simulink model "Problem1_model"  (R2016a)
settings: Solver=VariableStepAuto  StartTime=0.0  StopTime=10.0  RelTol=1e-3
values from neighbouring files (symbols this model uses):
  theta1_path = planTraj(x2_i(1),x2_f(1),time)    [Problem1.m]    (also in Problem2.m)
  theta2_path = planTraj(x2_i(2),x2_f(2),time)    [Problem1.m]    (also in Problem2.m)
undefined symbols (not defined in the file or in its folder): x2_i
settings Model: Creator=nathaniel  LastModifiedBy=nathaniel
settings GRTTargetCC: GeneratePreprocessorConditionals=Use local settings

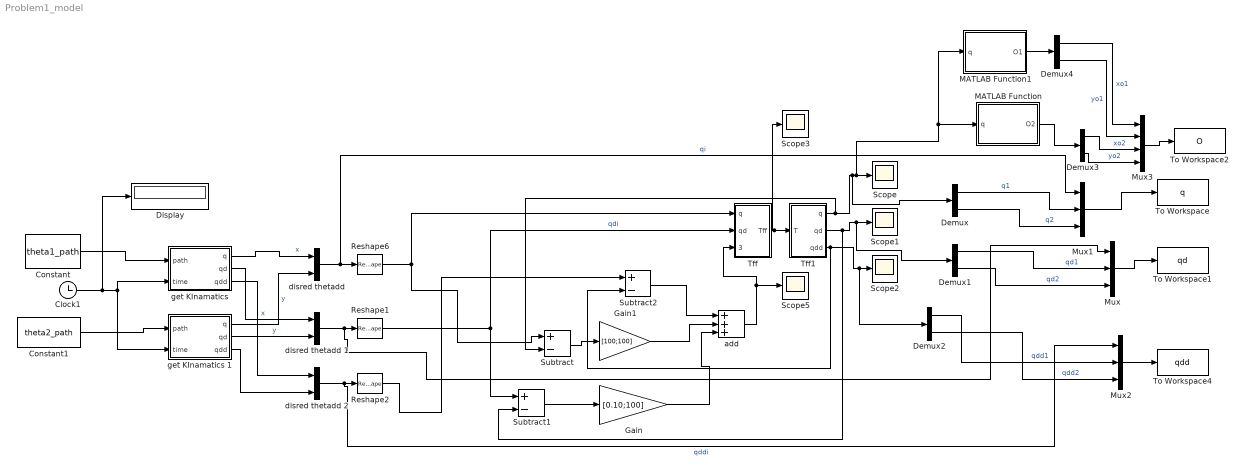
== system Problem1_model ==
  Clock1 : Clock
  Constant : Constant  Value=theta1_path
  Constant1 : Constant  Value=theta2_path
  Demux{,1..4} (5 alike) : Demux  Outputs=2
  Display : Display
  Gain : Gain  Gain=[0.10;100]
  Gain1 : Gain  Gain=[100;100]
  MATLAB Function : MATLAB Function  TreatAsAtomicUnit=on
  MATLAB Function1 : MATLAB Function  TreatAsAtomicUnit=on
  Mux : Mux  Inputs=3
  Mux1 : Mux  Inputs=3
  Mux2 : Mux  Inputs=3
  Mux3 : Mux
  Reshape1 : Reshape  OutputDimensionality=Column vector (2-D)
  Reshape2 : Reshape  OutputDimensionality=Column vector (2-D)
  Reshape6 : Reshape  OutputDimensionality=Column vector (2-D)
  Scope{,1..3,5} (5 alike) : Scope
  Subtract : Sum  Inputs=+-
  Subtract1 : Sum  Inputs=+-
  Subtract2 : Sum  Inputs=+-
  Tff : Subsystem
  Tff1 : Subsystem
  To Workspace : ToWorkspace  VariableName=q  SampleTime=-1
  To Workspace1 : ToWorkspace  VariableName=qd  SampleTime=-1
  To Workspace2 : ToWorkspace  VariableName=O  SampleTime=-1
  To Workspace4 : ToWorkspace  VariableName=qdd  SampleTime=-1
      settings: Save2DSignal=2-D array (concatenate along first dimension)
  "add " : Sum  Inputs=+++
  "disred thetadd " : Concatenate
  disred thetadd 1 : Concatenate
  disred thetadd 2 : Concatenate
  "get KInamatics " : MATLAB Function  TreatAsAtomicUnit=on
  get KInamatics 1 : MATLAB Function  TreatAsAtomicUnit=on
  wires:
  Clock1/1 -> Display/1, "get KInamatics "/2(time), get KInamatics 1/2(time)
  Constant1/1 -> get KInamatics 1/1(path)
  Constant/1 -> "get KInamatics "/1(path)
  Reshape1/1 -> Tff/2(qd), Subtract1/1  "qdi"
  Tff1/3(qdd) -> Subtract2/2, Demux2/1, Scope2/1
  Tff/1(Tff) -> Scope3/1, Tff1/1(T)
  Subtract/1 -> Gain1/1
  "add "/1 -> Scope5/1, Tff/3(qdd)
  Subtract1/1 -> Gain/1
  Gain1/1 -> "add "/2
  Reshape2/1 -> Subtract2/1
  Gain/1 -> "add "/3
  Reshape6/1 -> Tff/1(q), Subtract/1
  "disred thetadd "/1 -> Mux1/1, Reshape6/1  "qi"
  "get KInamatics "/1(q) -> "disred thetadd "/1  "x"
  get KInamatics 1/1(q) -> "disred thetadd "/2  "y"
  disred thetadd 1/1 -> Mux/1, Reshape1/1
  "get KInamatics "/2(qd) -> disred thetadd 1/1  "x"
  get KInamatics 1/2(qd) -> disred thetadd 1/2  "y"
  disred thetadd 2/1 -> Mux2/1, Reshape2/1  "qddi"
  "get KInamatics "/3(qdd) -> disred thetadd 2/1
  get KInamatics 1/3(qdd) -> disred thetadd 2/2
  Subtract2/1 -> "add "/1
  Tff1/1(q) -> Subtract/2, Demux/1, MATLAB Function1/1(q), MATLAB Function/1(q), Scope/1
  Demux/2 -> Mux1/3  "q2"
  Tff1/2(qd) -> Subtract1/2, Demux1/1, Scope1/1
  Mux/1 -> To Workspace1/1
  Demux1/1 -> Mux/2  "qd1"
  Demux1/2 -> Mux/3  "qd2"
  Demux/1 -> Mux1/2  "q1"
  Mux1/1 -> To Workspace/1
  Mux2/1 -> To Workspace4/1
  Demux2/1 -> Mux2/2  "qdd1"
  Demux2/2 -> Mux2/3  "qdd2"
  Demux3/2 -> Mux3/4  "yo2"
  Demux3/1 -> Mux3/3  "xo2"
  Mux3/1 -> To Workspace2/1
  MATLAB Function/1(O2) -> Demux3/1
  MATLAB Function1/1(O1) -> Demux4/1
  Demux4/1 -> Mux3/1  "xo1"
  Demux4/2 -> Mux3/2  "yo1"

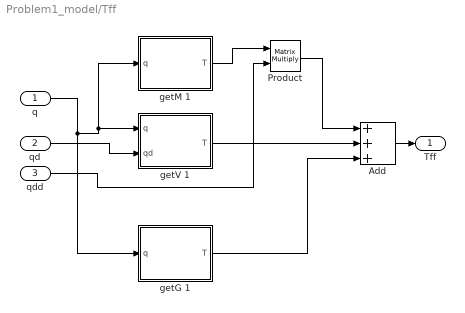
== system Problem1_model/Tff ==
  q : Inport
  qd : Inport  Port=2
  qdd : Inport  Port=3
  Add : Sum  Inputs=+++
  Product : Product  Multiplication=Matrix(*)
  getG 1 : MATLAB Function  TreatAsAtomicUnit=on
  getM 1 : MATLAB Function  TreatAsAtomicUnit=on
  getV 1 : MATLAB Function  TreatAsAtomicUnit=on
  Tff : Outport
  wires:
  q/1 -> getG 1/1(q), getV 1/1(q), getM 1/1(q)
  qdd/1 -> Product/2
  Add/1 -> Tff/1
  Product/1 -> Add/1
  getM 1/1(T) -> Product/1
  getG 1/1(T) -> Add/3
  qd/1 -> getV 1/2(qd)
  getV 1/1(T) -> Add/2

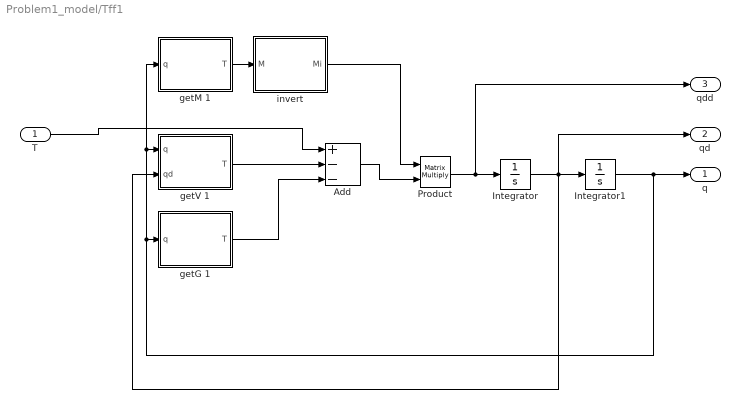
== system Problem1_model/Tff1 ==
  T : Inport
  Add : Sum  Inputs=+--
  Integrator : Integrator  InitialCondition=[0;0]
  Integrator1 : Integrator  InitialCondition=x2_i
  Product : Product  Multiplication=Matrix(*)
  getG 1 : MATLAB Function  TreatAsAtomicUnit=on
  getM 1 : MATLAB Function  TreatAsAtomicUnit=on
  getV 1 : MATLAB Function  TreatAsAtomicUnit=on
  invert : MATLAB Function  TreatAsAtomicUnit=on
  q : Outport
  qd : Outport  Port=2
  qdd : Outport  Port=3
  wires:
  getV 1/1(T) -> Add/2
  getG 1/1(T) -> Add/3
  T/1 -> Add/1
  getM 1/1(T) -> invert/1(M)
  invert/1(Mi) -> Product/1
  Add/1 -> Product/2
  Integrator/1 -> getV 1/2(qd), qd/1, Integrator1/1
  Integrator1/1 -> getM 1/1(q), getV 1/1(q), getG 1/1(q), q/1
  Product/1 -> qdd/1, Integrator/1

== matlab function Problem1_model/get KInamatics 1 ==
  data: path input; q output; time input; qd output; qdd output
function [ q,qd,qdd] = fcn(path, time)
%#codegen
[q qd qdd] = getKin(path, time);

== matlab function Problem1_model/get KInamatics  ==
  data: path input; q output; time input; qd output; qdd output
function [ q,qd,qdd] = fcn(path, time)
%#codegen
[q qd qdd] = getKin(path, time);

== matlab function Problem1_model/MATLAB Function ==
  data: q input; O2 output
function O2 = fcn(q)
%#codegen
a1 = 0.3;
a2 = 0.3
 O2 = getO2(a1,a2,q)

== matlab function Problem1_model/MATLAB Function1 ==
  data: q input; O1 output
function O1 = fcn(q)
%#codegen
a1 = 0.3;
a2 = 0.3
 O1 = getO1(a1,a2,q)

== matlab function Problem1_model/Tff/getM 1 ==
  data: q input; T output
function T = fcn(q)
%#codegen
T = getM(q);

== matlab function Problem1_model/Tff/getV 1 ==
  data: q input; T output; qd input
function T = fcn(q, qd)
%#codegen
T = getV(q, qd);

== matlab function Problem1_model/Tff/getG 1 ==
  data: q input; T output
function T = fcn(q)
%#codegen
T = getG(q);

== matlab function Problem1_model/Tff1/getG 1 ==
  data: q input; T output
function T = fcn(q)
%#codegen
T = getG(q);

== matlab function Problem1_model/Tff1/getM 1 ==
  data: q input; T output
function T = fcn(q)
%#codegen
T = getM(q);

== matlab function Problem1_model/Tff1/getV 1 ==
  data: q input; T output; qd input
function T = fcn(q, qd)
%#codegen
T = getV(q, qd);

== matlab function Problem1_model/Tff1/invert ==
  data: M input; Mi output
function Mi = fcn(M)
%#codegen
Mi =pinv(M);
